simulink model "Nicholas_DCAC_SineWaveInverter_noise"  (R2021b)
settings: Solver=VariableStepAuto  StartTime=0.0  StopTime=0.05  RelTol=1e-3  AbsTol=1e-3
libraries: spsDiodeLib x4, spsIGBTLib x4, spsSeriesRLCBranchLib x3, simulink x1, spsControlledVoltageSourceLib x1, spsDCVoltageSourceLib x1, spsGroundLib x1, spsMultimeterLib x1, spsTriangleGeneratorLib x1, spspowerguiLib x1
settings Model: Creator=cmr56  LastModifiedBy=NicholasYe
settings SolverCC: AutoScaleAbsTol=off  AlgebraicLoopSolver=TrustRegion
settings DebuggingCC: SymbolicDimsDataTypeCodeGenerationDiagnostic=none  SFMachineParentedDataDiag=warning
settings SFSimCC: CustomCodeUndefinedFunction=UseInterfaceOnly
settings SimscapeCC: SimscapeLogType=all  SimscapeLogSimulationStatistics=on  SimscapeLogDataHistory=10000

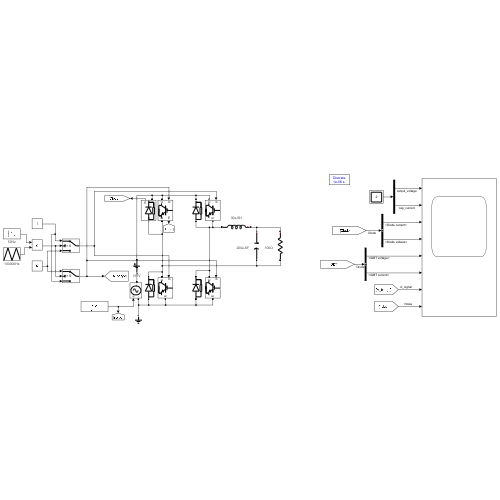
[thumbnail: Simulink's stored preview of the top-level diagram]
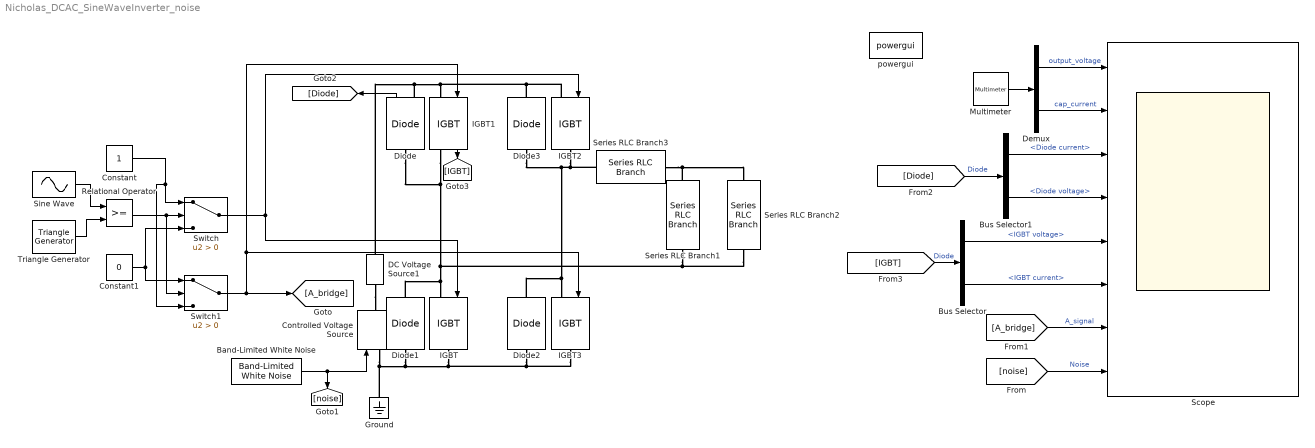
== system Nicholas_DCAC_SineWaveInverter_noise ==
  Band-Limited White Noise : simulink/Sources/Band-Limited White Noise  Cov=[0.05]  Ts=10e-4  seed=[23341]
  Bus Selector : BusSelector  OutputSignals=IGBT voltage,IGBT current
  Bus Selector1 : BusSelector  OutputSignals=Diode current,Diode voltage
  Constant : Constant
  Constant1 : Constant  Value=0
  Controlled Voltage Source : spsControlledVoltageSourceLib/Controlled Voltage Source  Initialize=on  Source_Type=AC  Amplitude=0  Phase=0  Frequency=0  Measurements=None
  DC Voltage Source1 : spsDCVoltageSourceLib/DC Voltage Source  Amplitude=311  Measurements=None
      settings: AttributesFormatString=%<Amplitude>V
  Demux : Demux  Outputs=2
  Diode : spsDiodeLib/Diode  Ron=0.001  Lon=0  Vf=0.8  IC=0  UseSnubber=0  Rs=500  Cs=250e-9  Measurements=on
  Diode1 : spsDiodeLib/Diode  Ron=0.001  Lon=0  Vf=0.8  IC=0  UseSnubber=0  Rs=500  Cs=250e-9  Measurements=off
  Diode2 : spsDiodeLib/Diode  Ron=0.001  Lon=0  Vf=0.8  IC=0  UseSnubber=0  Rs=500  Cs=250e-9  Measurements=off
  Diode3 : spsDiodeLib/Diode  Ron=0.001  Lon=0  Vf=0.8  IC=0  UseSnubber=0  Rs=500  Cs=250e-9  Measurements=off
  Ground : spsGroundLib/Ground  LConnTagsString=a
  IGBT : spsIGBTLib/IGBT  Ron=0.01  Lon=0  Vf=1  Tf=1e-6  Tt=2e-6  IC=0  Rs=1e5  Cs=inf  Measurements=off
  IGBT1 : spsIGBTLib/IGBT  Ron=0.01  Lon=0  Vf=1  Tf=1e-6  Tt=2e-6  IC=0  Rs=1e5  Cs=inf  Measurements=on
  IGBT2 : spsIGBTLib/IGBT  Ron=0.01  Lon=0  Vf=1  Tf=1e-6  Tt=2e-6  IC=0  Rs=1e5  Cs=inf  Measurements=off
  IGBT3 : spsIGBTLib/IGBT  Ron=0.01  Lon=0  Vf=1  Tf=1e-6  Tt=2e-6  IC=0  Rs=1e5  Cs=inf  Measurements=off
  Multimeter : spsMultimeterLib/Multimeter  PhasorSimulation=off  OutputType=Complex  sel=[1 3]  L=4  Gain=[1 1]  yselected={'Ub: Series RLC Branch1','Ib: Series RLC Branch1'};  PSBOutputType=1  PSBequivalent=0  AxesSetting=[0,0.1,-100,100]  Display=0  SavedBlockNames=-11
  Relational Operator : RelationalOperator  OutDataTypeStr=boolean  ZeroCross=off  RndMeth=Simplest
  Scope : Scope  NumInputPorts=8
  Series RLC Branch1 : spsSeriesRLCBranchLib/Series RLC Branch  LConnTagsString=__new0  RConnTagsString=__new0  BranchType=C  Resistance=1  Inductance=15e-6  SetiL0=off  InitialCurrent=0  Capacitance=200e-6  Setx0=off  InitialVoltage=0  Measurements=Branch voltage and current
      settings: AttributesFormatString=%<Capacitance>F
  Series RLC Branch2 : spsSeriesRLCBranchLib/Series RLC Branch  LConnTagsString=__new0  RConnTagsString=__new0  BranchType=R  Resistance=100  Inductance=15e-6  SetiL0=off  InitialCurrent=0  Capacitance=200e-6  Setx0=off  InitialVoltage=0  Measurements=None
      settings: AttributesFormatString=%<Resistance>Ω
  Series RLC Branch3 : spsSeriesRLCBranchLib/Series RLC Branch  LConnTagsString=__new0  RConnTagsString=__new0  BranchType=L  Resistance=1  Inductance=30e-6  SetiL0=off  InitialCurrent=0  Capacitance=100e-3  Setx0=off  InitialVoltage=0  Measurements=Branch voltage and current
      settings: AttributesFormatString=%<Inductance>H
  Sine Wave : Sin  Frequency=100*pi  SampleTime=0
      settings: AttributesFormatString=50Hz
  Switch : Switch  Criteria=u2 > Threshold
  Switch1 : Switch  Criteria=u2 > Threshold
  Triangle Generator : spsTriangleGeneratorLib/Triangle Generator  Freq=100000  Phase=0  Ts=0
      settings: AttributesFormatString=%<Freq>Hz
  powergui : spspowerguiLib/powergui  Priority=1  SimulationMode=Discrete  SampleTime=1e-8  frequency=60  Iterations=50  frequencyindice=0  Pbase=100e6  ErrMax=1e-4  UnitsV=kV  UnitsW=MW  buscounter=0  FunctionMessages=off  echomessages=off  EnableUseOfTLC=off  CurrentSourceSwitches=off  DisableSnubberDevices=off  DisableRonSwitches=off  DisableVfSwitches=off  DisplayEquations=off  AutomaticDiscreteSolvers=off  SolverType=Tustin/Backward Euler (TBE)  Interpol=off  ExternalGateDelay=off  methode=off  Ts=100  x0status=blocks  SPID=on  SwTol=0  HookPort=off  NonlinearTolerance=1e-4  nMaxIteration=100  ContinueOnMaxIteration=off  RestoreLinks=warning  ResistiveCurrentMeasurement=off  Frange=[0:2:500]  Ylog=off  Xlog=on  ShowGrid=off  save=off  variable=ZData  structure=0  ZoomFFT=off  StartTime=0.0  cycles=1  DisplayStyle=1  fundamental=60  FreqAxis=off  MaxFrequency=1000  frequencyindicesteady=1  RmsSteady=1  display=off
  wires:
  Sine Wave/1 -> Relational Operator/1
  Triangle Generator/1 -> Relational Operator/2
  Relational Operator/1 -> Switch1/2, Switch/2
  Constant1/1 -> Switch1/1, Switch/3
  Constant/1 -> Switch1/3, Switch/1
  Multimeter/1 -> Demux/1
  Switch1/1 -> IGBT3/1, IGBT1/1, [A_bridge]
  Switch/1 -> IGBT2/1, IGBT/1
  Demux/1 -> Scope/1  "output_voltage"
  Demux/2 -> Scope/2  "cap_current"
  [A_bridge] -> Scope/7  "A_signal"
  [noise] -> Scope/8  "Noise"
  IGBT1/1 -> [IGBT]
  Bus Selector/1 -> Scope/5  "<IGBT voltage>"
  Bus Selector/2 -> Scope/6  "<IGBT current>"
  Diode/1 -> [Diode]
  [Diode] -> Bus Selector1/1  "Diode"
  Bus Selector1/1 -> Scope/3  "<Diode current>"
  Bus Selector1/2 -> Scope/4  "<Diode voltage>"
  [IGBT] -> Bus Selector/1  "Diode"
  Band-Limited White Noise/1 -> Controlled Voltage Source/1, [noise]
  connections:
  IGBT/RConn1 -- Ground/LConn1 -- Controlled Voltage Source/LConn1 -- Diode1/LConn1 -- IGBT3/RConn1 -- Diode2/LConn1
  Diode/LConn1 -- IGBT1/RConn1 -- Series RLC Branch2/RConn1 -- Series RLC Branch1/RConn1 -- Diode1/RConn1 -- IGBT/LConn1
  DC Voltage Source1/RConn1 -- Diode/RConn1 -- Diode3/RConn1 -- IGBT2/LConn1 -- IGBT1/LConn1
  IGBT2/RConn1 -- Diode3/LConn1 -- Diode2/RConn1 -- IGBT3/LConn1 -- Series RLC Branch3/RConn1
  Series RLC Branch1/LConn1 -- Series RLC Branch3/LConn1 -- Series RLC Branch2/LConn1
  DC Voltage Source1/LConn1 -- Controlled Voltage Source/RConn1
